simulink subsystem "VehicleModel"  (R2023b)
settings: Solver=VariableStepAuto  StartTime=0.0  StopTime=10.0  RelTol=1e-3
undefined symbols (not defined in the file): EOL_Vehicle_Cf, EOL_Vehicle_Cr, EOL_Vehicle_INITR, EOL_Vehicle_InitX, EOL_Vehicle_InitY, EOL_Vehicle_Iz, EOL_Vehicle_lf, EOL_Vehicle_lr, EOL_Vehicle_M
settings Model: Creator=konur  LastModifiedBy=konur

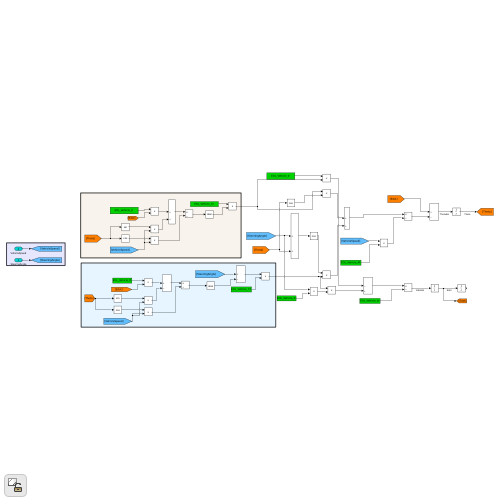
[thumbnail: Simulink's stored preview of the top-level diagram]
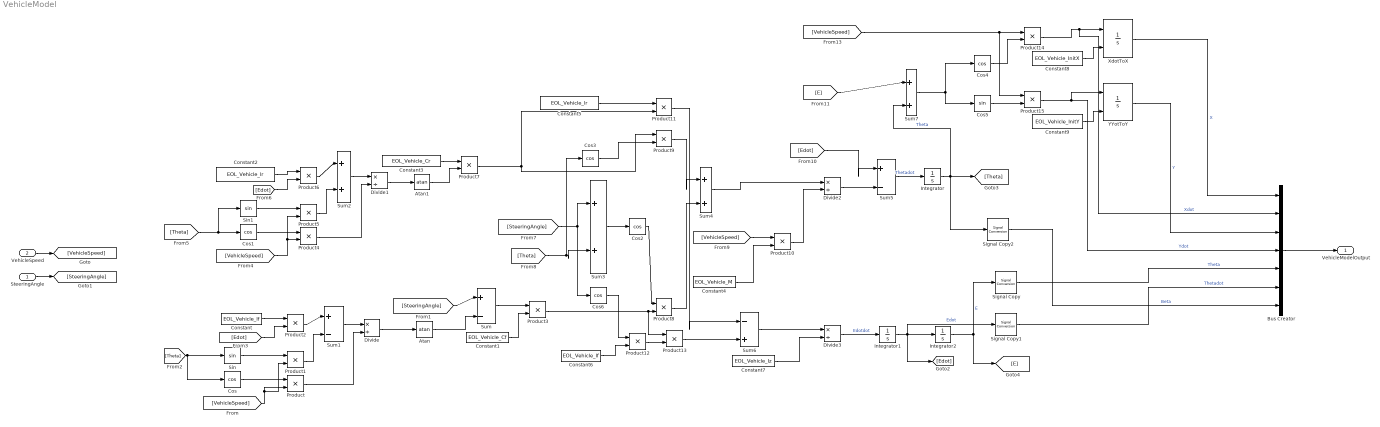
== system VehicleModel ==
  SteeringAngle : Inport  OutDataTypeStr=double
  VehicleSpeed : Inport  Port=2
  Atan : Trigonometry  Operator=atan  OutputSignalType=real
  Atan1 : Trigonometry  Operator=atan
  Bus Creator : BusCreator  Inputs=7  OutDataTypeStr=Bus: VehicleModelBus  NonVirtualBus=on
  Constant : Constant  Value=EOL_Vehicle_lf  OutDataTypeStr=double
  Constant1 : Constant  Value=EOL_Vehicle_Cf  OutDataTypeStr=double
  Constant2 : Constant  Value=EOL_Vehicle_lr  OutDataTypeStr=double
  Constant3 : Constant  Value=EOL_Vehicle_Cr  OutDataTypeStr=double
  Constant4 : Constant  Value=EOL_Vehicle_M  OutDataTypeStr=double
  Constant5 : Constant  Value=EOL_Vehicle_lr  OutDataTypeStr=double
  Constant6 : Constant  Value=EOL_Vehicle_lf  OutDataTypeStr=double
  Constant7 : Constant  Value=EOL_Vehicle_Iz  OutDataTypeStr=double
  Constant8 : Constant  Value=EOL_Vehicle_InitX  OutDataTypeStr=double
  Constant9 : Constant  Value=EOL_Vehicle_InitY  OutDataTypeStr=double
  Cos{,1..4,6} (6 alike) : Trigonometry  Operator=cos
  Cos5 : Trigonometry
  Divide{,1..3} (4 alike) : Product  Inputs=*/
  Integrator : Integrator
  Integrator1 : Integrator
  Integrator2 : Integrator  InitialCondition=EOL_Vehicle_INITR
  Product{,1..2,9,11} (5 alike) : Product
  Product{3..8,10,12..15} (11 alike) : Product  OutDataTypeStr=double
  Signal Copy : SignalConversion  OverrideOpt=off
  Signal Copy1 : SignalConversion  OverrideOpt=off
  Signal Copy2 : SignalConversion  OverrideOpt=off
  Sin : Trigonometry
  Sin1 : Trigonometry
  Sum : Sum  Inputs=|+-  OutDataTypeStr=double
  Sum1 : Sum  Inputs=|+-  OutDataTypeStr=double
  Sum2 : Sum  Inputs=|++  OutDataTypeStr=double
  Sum3 : Sum  Inputs=|++  OutDataTypeStr=double
  Sum4 : Sum  Inputs=|++  OutDataTypeStr=double
  Sum5 : Sum  Inputs=|+-  OutDataTypeStr=double
  Sum6 : Sum  Inputs=|-+  OutDataTypeStr=double  AccumDataTypeStr=double
  Sum7 : Sum  Inputs=|++  OutDataTypeStr=double  AccumDataTypeStr=double
  XdotToX : Integrator  InitialConditionSource=external  ContinuousStateAttributes='PositionX'
  YYotToY : Integrator  InitialConditionSource=external  ContinuousStateAttributes='PositionY'
  VehicleModelOutput : Outport  OutDataTypeStr=Bus: VehicleModelBus
  wires:
  Atan1/1 -> Product7/2
  Divide/1 -> Atan/1
  Product2/1 -> Sum1/1
  VehicleSpeed/1 -> [VehicleSpeed]
  [SteeringAngle] -> Sum/1
  Sum1/1 -> Divide/1
  Sum/1 -> Product3/1
  [Edot] -> Product2/2
  [VehicleSpeed] -> Product5/2, Product4/2
  [Theta] -> Sin1/1, Cos1/1
  [Edot] -> Product6/2
  Divide1/1 -> Atan1/1
  [Theta] -> Sin/1, Cos/1
  Cos/1 -> Product/1
  [VehicleSpeed] -> Product1/2, Product/2
  Product1/1 -> Sum1/2
  SteeringAngle/1 -> [SteeringAngle]
  Product/1 -> Divide/2
  Sin/1 -> Product1/1
  Atan/1 -> Sum/2
  Product5/1 -> Sum2/2
  Constant2/1 -> Product6/1
  Sin1/1 -> Product5/1
  Cos1/1 -> Product4/1
  Product4/1 -> Divide1/2
  Constant/1 -> Product2/1
  Constant1/1 -> Product3/2
  Product6/1 -> Sum2/1
  Sum2/1 -> Divide1/1
  Constant3/1 -> Product7/1
  [SteeringAngle] -> Sum3/1, Cos6/1
  [Theta] -> Cos3/1, Sum3/2
  Sum3/1 -> Cos2/1
  Cos2/1 -> Product8/1
  Product3/1 -> Product8/2, Product13/1
  Cos3/1 -> Product9/2
  Product7/1 -> Product11/2, Product9/1
  Product9/1 -> Sum4/1
  Product8/1 -> Sum4/2
  Sum4/1 -> Divide2/1
  Product10/1 -> Divide2/2
  Constant4/1 -> Product10/2
  [VehicleSpeed] -> Product10/1
  Divide2/1 -> Sum5/2
  Sum5/1 -> Integrator/1  "Thetadot"
  Integrator/1 -> [Theta], Signal Copy2/1, Sum7/2  "Theta"
  Constant5/1 -> Product11/1
  Constant6/1 -> Product12/2
  Product12/1 -> Product13/2
  Product13/1 -> Sum6/2
  Product11/1 -> Sum6/1
  Sum6/1 -> Divide3/1
  Constant7/1 -> Divide3/2
  Divide3/1 -> Integrator1/1  "Edotdot"
  Integrator1/1 -> [Edot], Integrator2/1, Signal Copy1/1  "Edot"
  [Edot] -> Sum5/1
  Sum7/1 -> Cos4/1, Cos5/1
  [E] -> Sum7/1
  [VehicleSpeed] -> Product14/1, Product15/1
  Cos4/1 -> Product14/2
  Product14/1 -> XdotToX/1, Bus Creator/2  "Xdot"
  XdotToX/1 -> Bus Creator/1  "X"
  Cos5/1 -> Product15/2
  Product15/1 -> YYotToY/1, Bus Creator/4  "Ydot"
  YYotToY/1 -> Bus Creator/3  "Y"
  Integrator2/1 -> [E], Signal Copy/1  "E"
  Cos6/1 -> Product12/1
  Constant8/1 -> XdotToX/2
  Constant9/1 -> YYotToY/2
  Signal Copy/1 -> Bus Creator/5  "Theta"
  Signal Copy1/1 -> Bus Creator/6  "Thetadot"
  Signal Copy2/1 -> Bus Creator/7  "Beta"
  Bus Creator/1 -> VehicleModelOutput/1
